simulink model "Jeos6DOF_IMU"  (R2022b)
settings: Solver=ode4  StartTime=0.0  StopTime=100  FixedStep=0.1  RelTol=1e-3
values from neighbouring files (symbols this model uses):
  a0_s2 = 0    [computeAeroForces.m]
  a0_s3 = 0    [computeAeroForces.m]
  a0_s4 = 0.05    [computeAeroForces.m]
  a0_s5 = 0.05    [computeAeroForces.m]
  AR_s2 = b_s2/c_s2    [computeSurfacePos.m]
  AR_s3 = b_s3/c_s3    [computeSurfacePos.m]
  AR_s4 = (b_s4 + b_s5)/c_s4    [computeSurfacePos.m]
  AR_s5 = (b_s4 + b_s5)/c_s5    [computeSurfacePos.m]
  area_s2 = c_s2 * b_s2    [computeSurfacePos.m]
  area_s3 = c_s3 * b_s3    [computeSurfacePos.m]
  area_s4 = c_s4 * b_s4    [computeSurfacePos.m]
  area_s5 = c_s5 * b_s5    [computeSurfacePos.m]
  c_s2 = componentMassesAndGeom(3,2)    [computeSurfacePos.m]
  c_s3 = componentMassesAndGeom(4,2)    [computeSurfacePos.m]
  c_s4 = componentMassesAndGeom(1,2)    [computeSurfacePos.m]
  c_s5 = componentMassesAndGeom(2,2)    [computeSurfacePos.m]
  CD0_s2 = 0.01    [computeAeroForces.m]
  CD0_s3 = 0.01    [computeAeroForces.m]
  CD0_s4 = 0.01    [computeAeroForces.m]
  CD0_s5 = 0.01    [computeAeroForces.m]
  CDa_s2 = 1    [computeAeroForces.m]
  CDa_s3 = 1    [computeAeroForces.m]
  CDa_s4 = 1    [computeAeroForces.m]
  CDa_s5 = 1    [computeAeroForces.m]
  CL0_s2 = 0    [computeAeroForces.m]
  CL0_s3 = 0    [computeAeroForces.m]
  CL0_s4 = 0.05    [computeAeroForces.m]
  CL0_s5 = 0.05    [computeAeroForces.m]
  CM0_s2 = 0    [computeAeroForces.m]
  CM0_s3 = 0    [computeAeroForces.m]
  CM0_s4 = -0.05    [computeAeroForces.m]
  CM0_s5 = -0.05    [computeAeroForces.m]
  CMa_s2 = 0    [computeAeroForces.m]
  CMa_s3 = 0    [computeAeroForces.m]
  CMa_s4 = 0    [computeAeroForces.m]
  CMa_s5 = 0    [computeAeroForces.m]
  e_s2 = 0.8    [computeAeroForces.m]
  e_s3 = 0.8    [computeAeroForces.m]
  e_s4 = 0.9    [computeAeroForces.m]
  e_s5 = 0.9    [computeAeroForces.m]
  i_s2 = 0    [computeAeroForces.m]
  i_s3 = 0    [computeAeroForces.m]
  i_s4 = 0.05    [computeAeroForces.m]
  i_s5 = 0.05    [computeAeroForces.m]
  Jxx = 1    [Sim_sixDOFdriverScript.m]
  Jxy = 0.    (= 0)    [Sim_sixDOFdriverScript.m]
  Jxz = 3    [Sim_sixDOFdriverScript.m]
  Jyx = 2    [Sim_sixDOFdriverScript.m]
  Jyy = 2    [Sim_sixDOFdriverScript.m]
  Jyz = 0    [Sim_sixDOFdriverScript.m]
  Jzx = Jxz    (= 3)    [Sim_sixDOFdriverScript.m]
  Jzy = Jyz    (= 0)    [Sim_sixDOFdriverScript.m]
  Jzz = 2    [Sim_sixDOFdriverScript.m]
  LL = 0.8    [Sim_sixDOFdriverScript.m]
  MM = 0.8    [Sim_sixDOFdriverScript.m]
  n_s2 = [0; 0; -1]    [computeAeroForces.m]
  n_s3 = [0; 1; 0]    [computeAeroForces.m]
  n_s4 = [0; 0; -1]    [computeAeroForces.m]
  n_s5 = [0; 0; -1]    [computeAeroForces.m]
  NN = 0.8    [Sim_sixDOFdriverScript.m]
  rEarth = 6378100    [Sim_sixDOFdriverScript.m]
  ro = 1.225    [computeAeroForces.m]
  x_S2_B_B = (x_S2_B_B_nominal + [0.25*c_s2 0 0]') - x_cg    [computeMassProps.m]
  x_S3_B_B = (x_S3_B_B_nominal + [0.25*c_s3 0 0]') - x_cg    [computeMassProps.m]
  x_S4_B_B = (x_S4_B_B_nominal + [0.25*c_s4 0 0]') - x_cg    [computeMassProps.m]
  x_S5_B_B = (x_S5_B_B_nominal + [0.25*c_s5 0 0]') - x_cg    [computeMassProps.m]
undefined symbols (not defined in the file or in its folder): earthRadius
libraries: simulink_extras x4, matrix_library x3, aerolibutil x2, sharedutil x1, simulink x1
(part 2 of 2)

== matlab function Jeos6DOF_IMU/JeoIMUmodel/TransKin_RotKin_TansDynam/Translational Kinematics/C_EN from LAX to ECEF ==
  data: lat input; ZYXDCM output; long input
function ZYXDCM = DCM_from_Euler(lat,long) % sequence of rotation is lat long
%     yaw_matrix = [cos(yaw) sin(yaw) 0;
%                   -sin(yaw) cos(yaw) 0;
%                   0 0 1];
    lat_matrix = [cos(lat) 0 -sin(lat);
                    0           1           0;
                    sin(lat) 0  cos(lat)];
    long_matrix = [1            0           0;
                    0          cos(-long)    sin(-long);
                    0           -sin(-long)  cos(-long)];

    adjust_matrix = [cos(pi/2) 0 -sin(pi/2);
                    0           1           0;
                    sin(pi/2) 0  cos(pi/2)];
    ZYXDCM = adjust_matrix*long_matrix*lat_matrix;
end

%this rotational matrix turns lat long coordinate into a new C_EN
%assuming the N CS is lat and longitudinally rotated, then you would do
%-longditudinal rotation then lat rotation, then rotate 90 degrees again to
%match ECEF

== matlab function Jeos6DOF_IMU/JeoIMUmodel/TransKin_RotKin_TansDynam/Rotational Kinematics_Euler/HinvMatrix ==
  data: pitchTheta input; hinv output; rollPhi input
function hinv = HinvMat(pitchTheta, rollPhi)
tThetasPhi = tan(pitchTheta) * sin(rollPhi);
tThetacPhi = tan(pitchTheta) * cos(rollPhi);
cPhi = cos(rollPhi);
sPhi = sin(rollPhi);
sPhiOvercTheta = sin(rollPhi)/cos(pitchTheta);
cPhiOvercTheta = cos(rollPhi)/cos(pitchTheta);

h = [1,tThetasPhi,tThetacPhi; 0,cPhi,-sPhi; 0,sPhiOvercTheta,cPhiOvercTheta];

hinv = h;

== matlab function Jeos6DOF_IMU/JeoIMUmodel/Rotational Kinematics_Strapdown/Omega_B_N ==
  data: P_degPs input; y output; Q_degPs input; R_degPs input
function y = Omega_B_N(P_degPs,Q_degPs,R_degPs)
% Function used to generate cross product matrix of body rates (P,Q,R)
% w.r.t NED. This is basically a skew symmetric matrix
Omega_B_N = [0,-R_degPs,Q_degPs; R_degPs,0,-P_degPs; -Q_degPs,P_degPs,0];
y = Omega_B_N;

== matlab function Jeos6DOF_IMU/JeoIMUmodel/Rotational Kinematics_Strapdown/dcmTOeuler ==
  data: inputDCM input; yaw_deg output; pitch_deg output; roll_deg output
function [yaw_deg, pitch_deg, roll_deg] = dcmTOEuler_TB(inputDCM)
% This function takes in a dcm and outputs the euler angles in a Tait-Bryan
% ZYX angle sequence
c12 = inputDCM(1,2);
c11 = inputDCM(1,1);
c13 = inputDCM(1,3);
c23 = inputDCM(2,3);
c33 = inputDCM(3,3);
yaw_deg = atand(c12/c11);
pitch_deg = -asind(c13);
roll_deg = atand(c23/c33);
end

== matlab function Jeos6DOF_IMU/JeoIMUmodel/Rotational Kinematics_Quaternions/quaternionMultiplication ==
  data: q1 input; qResult output; q2 input
function qResult = quaternionMultiplication(q1,q2)
q1imag = [q1(2); q1(3); q1(4)] ;
q2imag = [q2(2); q2(3); q2(4)];
qResultMag = q1(1)*q2(1) - dot(q1imag, q2imag);

qResultVect = q1(1)*q2imag + q2(1)*q1imag + cross(q1imag,q2imag);
qResult = [qResultMag; qResultVect];
end

== matlab function Jeos6DOF_IMU/JeoIMUmodel/Rotational Kinematics_Quaternions/quaternionToeuler ==
  data: qin input; yaw_deg output; pitch_deg output; roll_deg output
function [yaw_deg, pitch_deg, roll_deg] = quaternionsToEulerZYX(qin)
% Function to transfrom quaternion to Euler Angles in Tait-Bryan yaw,
% pitch, roll angle sequence

roll = atan2(2*(qin(1)*qin(2) + qin(3)*qin(4)), 1-2*(qin(2)^2 + qin(3)^2));
temp1 = sqrt(1+2*(qin(1)*qin(3)-qin(2)*qin(4)));
temp2 = sqrt(1-2*(qin(1)*qin(3) - qin(2)*qin(4)));
pitch = -pi/2 + 2*atan2(temp1, temp2);
yaw = atan2(2*(qin(1)*qin(4) + qin(2)*qin(3)) ,1-2*(qin(3)^2 + qin(4)^2));

yaw_deg = rad2deg(yaw);
pitch_deg = rad2deg(pitch);
roll_deg = rad2deg(roll);

end

== matlab function Jeos6DOF_IMU/JeoIMUmodel/Rotational Kinematics_Quaternions/NormalizeQuaternion ==
  data: qin input; qoutNorm output
function qoutNorm = NormalizeQuaternion(qin)
qinMag = norm(qin);
qoutNorm = qin/qinMag;

== matlab function Jeos6DOF_IMU/JeoIMUmodel/Rotational Dynamics/Using Cross Product Matrix/Omega Cross Matrix ==
  data: PQR input; omegaMat output
function omegaMat = fcn(PQR)
P = PQR(1); % deg
Q = PQR(2); % deg
R = PQR(3); % deg
omegaMat = [0 -R Q; R 0 -P; -Q P 0];

== matlab function Jeos6DOF_IMU/JeoIMUmodel/Aero Forces and Moments/F&M Horiz Stab Surface (S2)/Compute Aero Lift and Drag ==
  data: v_B_E_B input; alphaLocal output; v_B_A_B input; liftSurf output; dragSurf output; AR_s2 input; i_s2 input; n_s2 input; CL0_s2 input; CD0_s2 input; CDa_s2 input; a0_s2 input; e_s2 input; ro input; area_s2 input
function [alphaLocal, liftSurf, dragSurf] = fcn(v_B_E_B, v_B_A_B, AR_s2, i_s2, n_s2, CL0_s2, CD0_s2, CDa_s2, a0_s2, e_s2, ro, area_s2)
% Compute the lift and drag forces at the respective surface
% arSurf -> Aspect Ratio of respective surfaace
% ro -> air density (note: varies with altitude)
% v_infSurf -> total airspeed at the surface, i.e. Velocity of body w.r.t Inertial/ECEF as
% measured in body frame (|V_B_E_B|)
% v_B_A_B -> relative airspeed, where it is typically 
% v_B_E_B - c_B_N * v_A_N_N and v_A_N_N is the velocity of air mass w.r.t. NED 
% nSurf_B -> Normal force applied at surface
% eSurf -> Oswald efficiency
% alphaLocal0 -> Minimum drag Angle of Attack

v_infSurf = norm(v_B_E_B);
cSurfLocAlpha = 2*pi * (AR_s2/(2+AR_s2)); % Lift coefficient at the respective surface due to the local alpha (Angle of Attack)
alphaLocal = i_s2 - asin(dot(v_B_A_B,n_s2)/norm(v_B_A_B)); % in Radians
cSurfLift = CL0_s2 + cSurfLocAlpha * alphaLocal; % Lift coefficient of surface
cSurfDrag = CD0_s2 + CDa_s2 *(alphaLocal - a0_s2)^2 + (cSurfLift^2/(pi*e_s2*AR_s2));

liftSurf = cSurfLift * 0.5 * ro * (v_infSurf^2)*area_s2;
dragSurf = cSurfDrag * 0.5 * ro * (v_infSurf^2)*area_s2;
